simulink model "simRobotControlSystem_fixGap"  (R2016b)
settings: Solver=VariableStepAuto  StartTime=0.0  StopTime=10.0  RelTol=1e-3
undefined symbols (not defined in the file): Accelerations, Positions, TimeFromStart, Velocities
libraries: robotlib x3
settings Model: Creator=PC15  LastModifiedBy=PC15

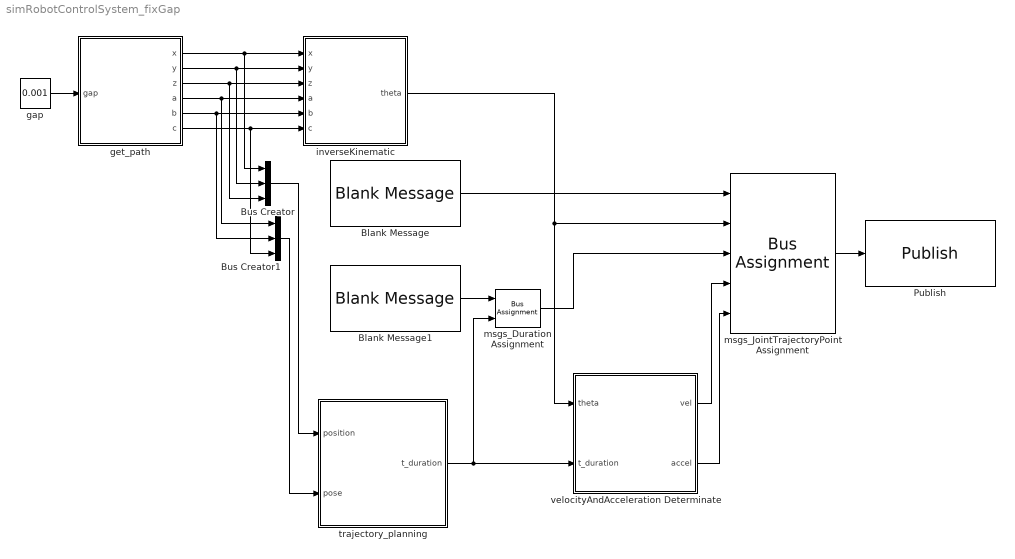
== system simRobotControlSystem_fixGap ==
  Blank Message : robotlib/Blank Message  SourceLibraryInfo=This block requires Robotics System Toolbox  messageType=trajectory_msgs/JointTrajectoryPoint  SampleTime=inf
  Blank Message1 : robotlib/Blank Message  SourceLibraryInfo=This block requires Robotics System Toolbox  messageType=std_msgs/Duration  SampleTime=inf
  Bus Creator : BusCreator  Inputs='x','y','z'
  Bus Creator1 : BusCreator  Inputs='a','b','c'
  Publish : robotlib/Publish  SourceLibraryInfo=This block requires Robotics System Toolbox  topicSource=Specify your own  topic=/trajectory_topic  messageType=trajectory_msgs/JointTrajectoryPoint  messageQueueLength=1
  gap : Constant  Value=0.001
  get_path : MATLAB Function  TreatAsAtomicUnit=on
  inverseKinematic : MATLAB Function  TreatAsAtomicUnit=on
  msgs_Duration Assignment : BusAssignment  AssignedSignals=Data.Sec
  msgs_JointTrajectoryPoint Assignment : BusAssignment  AssignedSignals=Positions,TimeFromStart,Velocities,Accelerations
  trajectory_planning : MATLAB Function  TreatAsAtomicUnit=on
  velocityAndAcceleration Determinate : MATLAB Function  TreatAsAtomicUnit=on
  wires:
  get_path/6(c) -> inverseKinematic/6(c), Bus Creator1/3
  get_path/1(x) -> Bus Creator/1, inverseKinematic/1(x)
  get_path/4(a) -> Bus Creator1/1, inverseKinematic/4(a)
  get_path/3(z) -> Bus Creator/3, inverseKinematic/3(z)
  get_path/5(b) -> Bus Creator1/2, inverseKinematic/5(b)
  get_path/2(y) -> Bus Creator/2, inverseKinematic/2(y)
  Bus Creator/1 -> trajectory_planning/1(position)
  Bus Creator1/1 -> trajectory_planning/2(pose)
  Blank Message1/1 -> msgs_Duration Assignment/1
  trajectory_planning/1(t_duration) -> msgs_Duration Assignment/2, velocityAndAcceleration Determinate/2(t_duration)
  Blank Message/1 -> msgs_JointTrajectoryPoint Assignment/1
  inverseKinematic/1(theta) -> velocityAndAcceleration Determinate/1(theta), msgs_JointTrajectoryPoint Assignment/2
  msgs_Duration Assignment/1 -> msgs_JointTrajectoryPoint Assignment/3
  msgs_JointTrajectoryPoint Assignment/1 -> Publish/1
  velocityAndAcceleration Determinate/1(vel) -> msgs_JointTrajectoryPoint Assignment/4
  velocityAndAcceleration Determinate/2(accel) -> msgs_JointTrajectoryPoint Assignment/5
  gap/1 -> get_path/1(gap)

== matlab function simRobotControlSystem_fixGap/get_path ==
  data: x output; gap input; y output; z output; a output; b output; c output
function [x,y,z,a,b,c] = path_fcn(gap)
u=0:gap:1;
[x,y,z] = line_function1(u);
[a,b,c] = line_function1(u,'pose');

end

== matlab function simRobotControlSystem_fixGap/inverseKinematic ==
  data: x input; theta output; y input; z input; a input; b input; c input
function theta  = inverseKinematic(x,y,z,a,b,c)

theta = [theta1;theta2;theta3;theta4;theta5;theta6];

== matlab function simRobotControlSystem_fixGap/trajectory_planning ==
  data: t_duration output; position input; pose input
function t_duration   = trajectory_planning( position,pose)

t_duration = u;

end

== matlab function simRobotControlSystem_fixGap/velocityAndAcceleration Determinate ==
  data: theta input; vel output; t_duration input; accel output
function [vel,accel] = velAndAccel_calculation(theta,t_duration)

vel=u;
accel=u;
end
